simulink model "SEPIC_PhysicalModel_FMU"  (R2024b)
settings: Solver=VariableStepAuto  StartTime=0.0  StopTime=10.0  RelTol=1e-3
undefined symbols (not defined in the file): D1_Vf, FPWM1, FPWM1_Volt, M1_Vth, PR1_Res, psu_V, R9_Res
libraries: fl_lib x10, ee_lib x8, nesl_utility x7, simulink x1
settings Model: DataDictionary=GlobalDataD_SEPIC_PhysicalCircuit.sldd  ExtModeTrigDuration=100  Creator=vlenzi  LastModifiedBy=vlenzi
settings DataIOCC: StateSaveName=tmp_raccel_xout
settings OptimizationCC: EfficientMapNaN2IntZero=off
settings DebuggingCC: ModelReferenceSymbolNameMessage=none
settings HardwareCC: TargetBitPerPointer=64  TargetBitPerSizeT=64  TargetBitPerPtrDiffT=64  TargetLongLongMode=on  TargetIntDivRoundTo=Zero  TargetEndianess=LittleEndian  TargetWordSize=64  TargetHWDeviceType=MATLAB Host  ProdEqTarget=off
settings RTWCC: SystemTargetFile=raccel.tlc  TemplateMakefile=raccel_default_tmf  RTWVerbose=off  RTWUseSimCustomCode=on  CustomBLASCallback=coder.internal.blas.MATLABBLASCallback
settings CodeAppCC: GenerateComments=off  MaxIdLength=128  MangleLength=10  SimulinkBlockComments=off
settings RaccelTargetCC: TargetLangStandard=C99 (ISO)  InstructionSetFMA=off  OptimizeReductions=off  LogToMDFFile=off  ENABLE_SLEXEC_SSBRIDGE=1  RTWCAPIParams=on  RTWCAPIRootIO=on

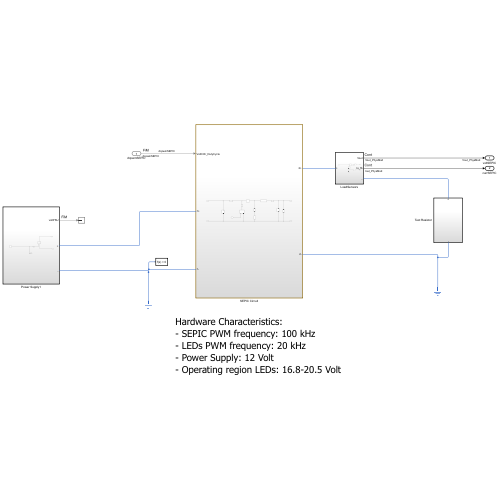
[thumbnail: Simulink's stored preview of the top-level diagram]
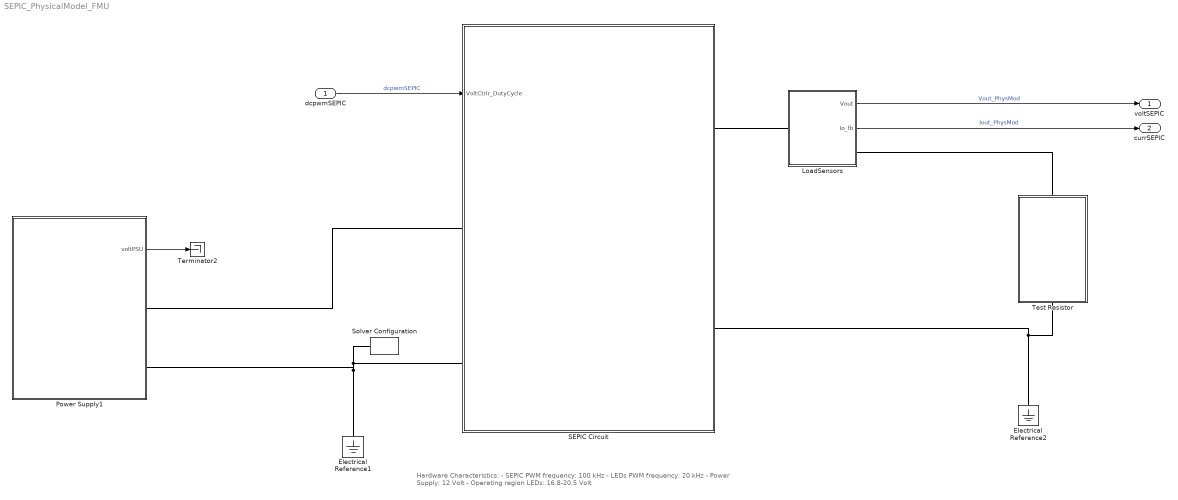
== system SEPIC_PhysicalModel_FMU ==
  note: Hardware Characteristics:
      | - SEPIC PWM frequency: 100 kHz
      | - LEDs PWM frequency: 20 kHz
      | - Power Supply: 12 Volt
      | - Operating region LEDs: 16.8-20.5 Volt
  dcpwmSEPIC : Inport  OutDataTypeStr=double  Unit=1  PortDimensions=1
  Electrical Reference1 : fl_lib/Electrical/Electrical Elements/Electrical Reference
  Electrical Reference2 : fl_lib/Electrical/Electrical Elements/Electrical Reference
  LoadSensors : Subsystem
  Power Supply1 : Subsystem  VariantControl=PowerSupply
  SEPIC Circuit : Subsystem
  Solver Configuration : nesl_utility/Solver Configuration  PhysicalDomain=network_engine_domain  SubClassName=solver  LeftPortType=input  RightPortType=generic  Tones=[]  Harmonics=[]  SimulateNoise=off  Profile=off  UseLocalSampling=off  EnableSwitchedLinearOptims=on  FrequencyDomain=off  UseCCode=off  RelTol=0.001  AbsTol=1e-06  MinStep=1e-09  ToWorkspace=off  RevertToSquareIcSolve=off  NumHomotopyIterations=100  PhasorMode=off  PhasorModeNumHarmonics=1  ConsistencySolver=NEWTON_XTOL_AFTER_FTOL  IndexReductionMethod=DerivativeReplacement  DoDC=off  ResidualTolerance=1e-9  ConsistencyTolSource=GLOBAL  ConsistencyAbsTol=0.001  ConsistencyRelTol=0.001  ConsistencyTolFactor=0.001  UseLocalSolver=off  LocalSolverChoice=NE_BACKWARD_EULER_ADVANCER  ResolveIndetEquations=on  FunctionEvalNumThread=1  LocalSolverSampleTime=2e-7  DoFixedCost=off  MaxNonlinIter=2  MaxModeIter=2  ComputeImpulses=off  ImpulseIterations=2  LinearAlgebra=Sparse  LinearAlgebraNumThread=0  EquationFormulation=NE_TIME_EF  DelaysMemoryBudget=1024  AutomaticFiltering=on  FilteringTimeConstant=0.001  PartitionStorageMethod=AS_NEEDED  PartitionMemoryBudget=1024  PartitionMethod=ROBUST  MultibodyUseLocalSolver=off  MultibodyLocalSolverChoice=ODE1  MultibodyLocalSolverSampleTime=0.001
  Terminator2 : Terminator
  Test Resistor : Subsystem  VariantControl=Resistor
  voltSEPIC : Outport  OutDataTypeStr=double  Unit=V  PortDimensions=1  VectorParamsAs1DForOutWhenUnconnected=off
  currSEPIC : Outport  Port=2  OutDataTypeStr=double  Unit=mA  PortDimensions=1  VectorParamsAs1DForOutWhenUnconnected=off
  wires:
  dcpwmSEPIC/1 -> SEPIC Circuit/1(VoltCtrlr_DutyCycle)  "dcpwmSEPIC"
  LoadSensors/1(Vout) -> voltSEPIC/1  "Vout_PhysMod"
  Power Supply1/1(voltPSU) -> Terminator2/1
  LoadSensors/2(Io_fb) -> currSEPIC/1  "Iout_PhysMod"
  connections:
  Power Supply1/RConn1 -- SEPIC Circuit/LConn1
  Solver Configuration/RConn1 -- Power Supply1/RConn2 -- Electrical Reference1/LConn1 -- SEPIC Circuit/LConn2
  SEPIC Circuit/RConn1 -- LoadSensors/LConn1
  Electrical Reference2/LConn1 -- SEPIC Circuit/RConn2 -- Test Resistor/RConn1
  Test Resistor/LConn1 -- LoadSensors/RConn1

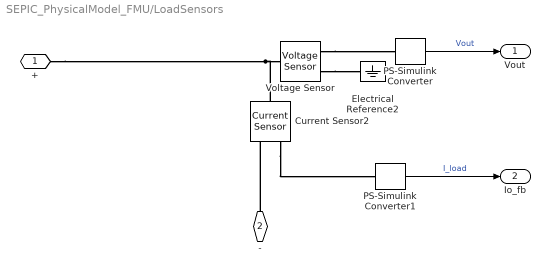
== system SEPIC_PhysicalModel_FMU/LoadSensors ==
  Current Sensor2 : fl_lib/Electrical/Electrical Sensors/Current Sensor
  Electrical Reference2 : fl_lib/Electrical/Electrical Elements/Electrical Reference
  PS-Simulink Converter : nesl_utility/PS-Simulink Converter  PhysicalDomain=network_engine_domain  SubClassName=ps_output  LeftPortType=input  RightPortType=output  PseudoPeriodic=off  Frequencies=[]  VectorFormat=1-D array  Unit=V  AffineConversion=off
  PS-Simulink Converter1 : nesl_utility/PS-Simulink Converter  PhysicalDomain=network_engine_domain  SubClassName=ps_output  LeftPortType=input  RightPortType=output  PseudoPeriodic=off  Frequencies=[]  VectorFormat=1-D array  Unit=mA  AffineConversion=off
  Voltage Sensor : fl_lib/Electrical/Electrical Sensors/Voltage Sensor
  + : PMIOPort  Side=Left
  - : PMIOPort  Port=2  Side=Right
  Vout : Outport  VectorParamsAs1DForOutWhenUnconnected=off
  Io_fb : Outport  Port=2  VectorParamsAs1DForOutWhenUnconnected=off
  wires:
  PS-Simulink Converter1/1 -> Io_fb/1  "I_load"
  PS-Simulink Converter/1 -> Vout/1  "Vout"
  connections:
  Voltage Sensor/RConn1 -- PS-Simulink Converter/LConn1
  Voltage Sensor/RConn2 -- Electrical Reference2/LConn1
  Current Sensor2/LConn1 -- Voltage Sensor/LConn1 -- +/RConn1
  Current Sensor2/RConn1 -- PS-Simulink Converter1/LConn1
  -/RConn1 -- Current Sensor2/RConn2

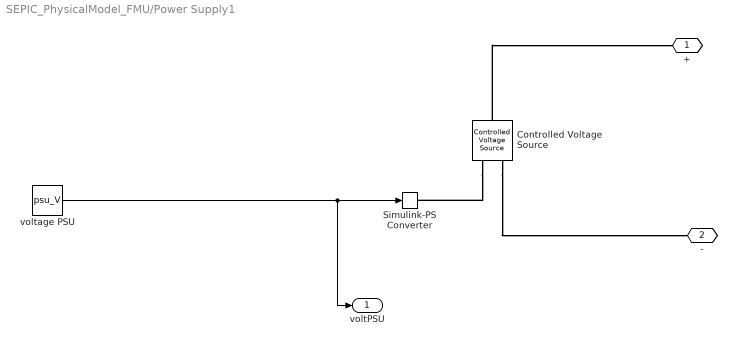
== system SEPIC_PhysicalModel_FMU/Power Supply1 ==
  Controlled Voltage Source : fl_lib/Electrical/Electrical Sources/Controlled Voltage Source
  Simulink-PS Converter : nesl_utility/Simulink-PS Converter  PhysicalDomain=network_engine_domain  SubClassName=ps_input  LeftPortType=input  RightPortType=output  PseudoPeriodic=off  Frequencies=[]  NoiseDistribution=none  NoiseParameters=[]  Unit=V  AffineConversion=off  FilteringAndDerivatives=filter  SimscapeFilterOrder=1  InputFilterTimeConstant=0.001  UdotUserProvided=0
  voltage PSU : Constant  Value=psu_V  OutDataTypeStr=double  SampleTime=-1
  + : PMIOPort  Side=Right
  - : PMIOPort  Port=2  Side=Right
  voltPSU : Outport  Unit=V  VectorParamsAs1DForOutWhenUnconnected=off
  wires:
  voltage PSU/1 -> voltPSU/1, Simulink-PS Converter/1
  connections:
  Controlled Voltage Source/RConn2 -- -/RConn1
  Controlled Voltage Source/RConn1 -- Simulink-PS Converter/RConn1
  Controlled Voltage Source/LConn1 -- +/RConn1

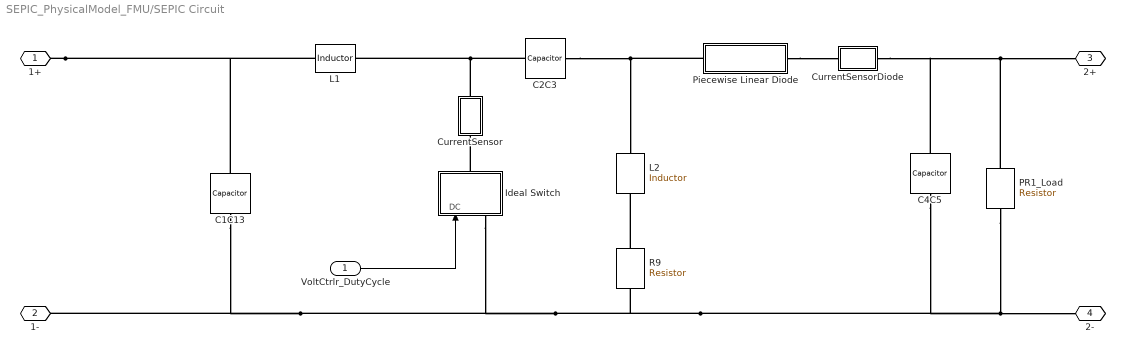
== system SEPIC_PhysicalModel_FMU/SEPIC Circuit ==
  VoltCtrlr_DutyCycle : Inport  Unit=1  PortDimensions=1
  C1C13 : ee_lib/Passive/Capacitor  cap_option=ee.enum.passive.capacitor.capOption.const  c=C1C13_Cap uF  Cvec=[1e-05, 1e-06] F  Vvec=[0, 10] V  CV_table_symmetry=1  f_vec=[1, 10] kHz  DFext_vec=[.8, 1.2]  enable_C_tol=0  averaging_period=0 s  C_tol=C1C13_Tol  tol_distribution=1  nSigma=4  r=1e-6 Ohm  g=0 1/Ohm  enable_operating_limits=0  operating_limit_action=2  max_working_voltage_range=[-25, 25] V  power_rating=1 W  maxTemperature=85 degC  thermalEnable=false  thermalMass=1 J/K  fault_action=simscape.enum.assert.action.none  t_fault=1 s  i_specify=off  i_priority=None  i=0 A  i_nominal_specify=off  i_nominal_value=1  i_nominal_unit=A  v_specify=off  v_priority=High  v=psu_V V  v_nominal_specify=off  v_nominal_value=1  v_nominal_unit=V  vc_specify=off  vc_priority=High  vc=psu_V V  vc_nominal_specify=off  vc_nominal_value=1  vc_nominal_unit=V  T_specify=off  T_priority=None  T=298.15 K  T_nominal_specify=off  T_nominal_value=1  T_nominal_unit=K
  C2C3 : ee_lib/Passive/Capacitor  cap_option=ee.enum.passive.capacitor.capOption.const  c=C2C3_Cap uF  Cvec=[1e-05, 1e-06] F  Vvec=[0, 10] V  CV_table_symmetry=1  f_vec=[1, 10] kHz  DFext_vec=[.8, 1.2]  enable_C_tol=0  averaging_period=0 s  C_tol=C2C3_Tol  tol_distribution=1  nSigma=4  r=1e-6 Ohm  g=0 1/Ohm  enable_operating_limits=0  operating_limit_action=2  max_working_voltage_range=[-25, 25] V  power_rating=1 W  maxTemperature=85 degC  thermalEnable=false  thermalMass=1 J/K  fault_action=simscape.enum.assert.action.none  t_fault=1 s  i_specify=off  i_priority=None  i=0 A  i_nominal_specify=off  i_nominal_value=1  i_nominal_unit=A  v_specify=off  v_priority=High  v=psu_V V  v_nominal_specify=off  v_nominal_value=1  v_nominal_unit=V  vc_specify=off  vc_priority=High  vc=psu_V V  vc_nominal_specify=off  vc_nominal_value=1  vc_nominal_unit=V  T_specify=off  T_priority=None  T=298.15 K  T_nominal_specify=off  T_nominal_value=1  T_nominal_unit=K
  C4C5 : ee_lib/Passive/Capacitor  cap_option=ee.enum.passive.capacitor.capOption.const  c=C4C5_Cap uF  Cvec=[1e-05, 1e-06] F  Vvec=[0, 10] V  CV_table_symmetry=1  f_vec=[1, 10] kHz  DFext_vec=[.8, 1.2]  enable_C_tol=0  averaging_period=0 s  C_tol=C4C5_Tol  tol_distribution=1  nSigma=4  r=1e-6 Ohm  g=0 1/Ohm  enable_operating_limits=0  operating_limit_action=2  max_working_voltage_range=[-25, 25] V  power_rating=1 W  maxTemperature=85 degC  thermalEnable=false  thermalMass=1 J/K  fault_action=simscape.enum.assert.action.none  t_fault=1 s  i_specify=off  i_priority=None  i=0 A  i_nominal_specify=off  i_nominal_value=1  i_nominal_unit=A  v_specify=off  v_priority=High  v=desiredVoltage_Param V  v_nominal_specify=off  v_nominal_value=1  v_nominal_unit=V  vc_specify=off  vc_priority=High  vc=desiredVoltage_Param V  vc_nominal_specify=off  vc_nominal_value=1  vc_nominal_unit=V  T_specify=off  T_priority=None  T=298.15 K  T_nominal_specify=off  T_nominal_value=1  T_nominal_unit=K
  CurrentSensor : Subsystem
  CurrentSensorDiode : Subsystem
  Ideal Switch : Subsystem  VariantControl=Ideal
  L1 : ee_lib/Passive/Inductor  l=L1_Ind uH  enable_L_tol=0  L_tol=L1_Tol  tol_distribution=1  nSigma=4  r=L1_Res Ohm  g=0 1/Ohm  enable_operating_limits=0  operating_limit_action=2  max_working_current=1 A  power_rating=1 W  fault_action=simscape.enum.assert.action.none  t_fault=1 s  i_L_specify=off  i_L_priority=High  i_L=0 A  i_L_nominal_specify=off  i_L_nominal_value=1  i_L_nominal_unit=A
  L2 : ee_lib/Passive/Inductor  l=L2_Ind uH  enable_L_tol=0  L_tol=L2_Tol  tol_distribution=1  nSigma=4  r=L2_Res Ohm  g=0 1/Ohm  enable_operating_limits=0  operating_limit_action=2  max_working_current=1 A  power_rating=1 W  fault_action=simscape.enum.assert.action.none  t_fault=1 s  i_L_specify=off  i_L_priority=High  i_L=0 A  i_L_nominal_specify=off  i_L_nominal_value=1  i_L_nominal_unit=A
  PR1_Load : ee_lib/Passive/Resistor  R=PR1_Res Ohm  enable_R_tol=0  R_tol=PR1_Tol  tol_distribution=1  nSigma=4  enable_operating_limits=0  operating_limit_action=2  power_rating=1 W  max_working_voltage=100 V  noise_mode=0  Tdevice=25 degC  sample_time=1e-3 s  repeatability=1  user_seed=0  auto_seed=1185518679  fault_action=simscape.enum.assert.action.none  t_fault=1 s  power_derating_T1=70 degC  power_derating_T2=155 degC  operating_temperature_range_vec=[-50, 150] degC  alpha=3.93e-3 1/K  Tmeas=25 degC  thermal_mass=100 J/K  temperature_specify=off  temperature_priority=High  temperature=298.15 K  temperature_nominal_specify=off  temperature_nominal_value=1  temperature_nominal_unit=K
  Piecewise Linear Diode : Subsystem  VariantControl=PiecewiseLinear
  R9 : ee_lib/Passive/Resistor  R=R9_Res Ohm  enable_R_tol=2  R_tol=R9_Tol  tol_distribution=1  nSigma=4  enable_operating_limits=0  operating_limit_action=2  power_rating=1 W  max_working_voltage=100 V  noise_mode=0  Tdevice=25 degC  sample_time=1e-3 s  repeatability=1  user_seed=0  auto_seed=2919300768  fault_action=simscape.enum.assert.action.none  t_fault=1 s  power_derating_T1=70 degC  power_derating_T2=155 degC  operating_temperature_range_vec=[-50, 150] degC  alpha=3.93e-3 1/K  Tmeas=25 degC  thermal_mass=100 J/K  temperature_specify=off  temperature_priority=High  temperature=298.15 K  temperature_nominal_specify=off  temperature_nominal_value=1  temperature_nominal_unit=K
  1+ : PMIOPort  Side=Left
  1- : PMIOPort  Port=2  Side=Left
  2+ : PMIOPort  Port=3  Side=Right
  2- : PMIOPort  Port=4  Side=Right
  wires:
  VoltCtrlr_DutyCycle/1 -> Ideal Switch/1(DC)
  connections:
  C2C3/LConn1 -- L1/RConn1 -- CurrentSensor/LConn1
  PR1_Load/LConn1 -- 2+/RConn1 -- CurrentSensorDiode/RConn1 -- C4C5/LConn1
  C2C3/RConn1 -- Piecewise Linear Diode/LConn1 -- L2/LConn1
  PR1_Load/RConn1 -- 2-/RConn1 -- C4C5/RConn1 -- R9/RConn1 -- Ideal Switch/LConn1 -- 1-/RConn1 -- C1C13/RConn1
  1+/RConn1 -- C1C13/LConn1 -- L1/LConn1
  Ideal Switch/RConn1 -- CurrentSensor/RConn1
  R9/LConn1 -- L2/RConn1
  Piecewise Linear Diode/RConn1 -- CurrentSensorDiode/LConn1

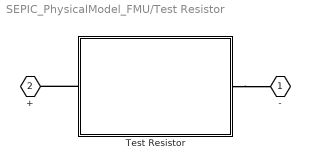
== system SEPIC_PhysicalModel_FMU/Test Resistor ==
  Test Resistor : Subsystem  VariantControl=Resistor  mask(Test Resistor){R_load=101.1, R_tol=1}
      mask prompts: R_load "Load Resistance [ohm]"; R_tol "Tolerance [%]"
      mask help: Test resistor with Load in the name, so that it can be triggered by ee_getEfficiency function.
  - : PMIOPort  Side=Right
  + : PMIOPort  Port=2  Side=Left
  connections:
  Test Resistor/LConn1 -- +/RConn1
  Test Resistor/RConn1 -- -/RConn1

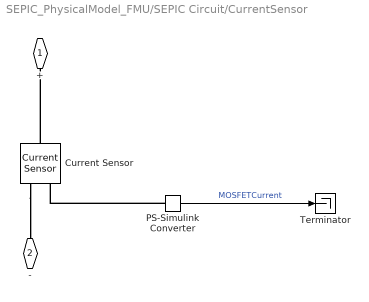
== system SEPIC_PhysicalModel_FMU/SEPIC Circuit/CurrentSensor ==
  Current Sensor : fl_lib/Electrical/Electrical Sensors/Current Sensor
  PS-Simulink Converter : nesl_utility/PS-Simulink Converter  PhysicalDomain=network_engine_domain  SubClassName=ps_output  LeftPortType=input  RightPortType=output  PseudoPeriodic=off  Frequencies=[]  VectorFormat=1-D array  Unit=A  AffineConversion=off
  Terminator : Terminator
  + : PMIOPort  Side=Left
  - : PMIOPort  Port=2  Side=Right
  wires:
  PS-Simulink Converter/1 -> Terminator/1  "MOSFETCurrent"
  connections:
  Current Sensor/LConn1 -- +/RConn1
  PS-Simulink Converter/LConn1 -- Current Sensor/RConn1
  Current Sensor/RConn2 -- -/RConn1

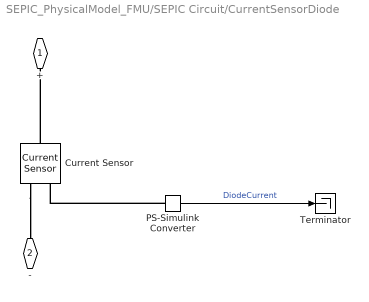
== system SEPIC_PhysicalModel_FMU/SEPIC Circuit/CurrentSensorDiode ==
  Current Sensor : fl_lib/Electrical/Electrical Sensors/Current Sensor
  PS-Simulink Converter : nesl_utility/PS-Simulink Converter  PhysicalDomain=network_engine_domain  SubClassName=ps_output  LeftPortType=input  RightPortType=output  PseudoPeriodic=off  Frequencies=[]  VectorFormat=1-D array  Unit=A  AffineConversion=off
  Terminator : Terminator
  + : PMIOPort  Side=Left
  - : PMIOPort  Port=2  Side=Right
  wires:
  PS-Simulink Converter/1 -> Terminator/1  "DiodeCurrent"
  connections:
  Current Sensor/RConn2 -- -/RConn1
  PS-Simulink Converter/LConn1 -- Current Sensor/RConn1
  Current Sensor/LConn1 -- +/RConn1

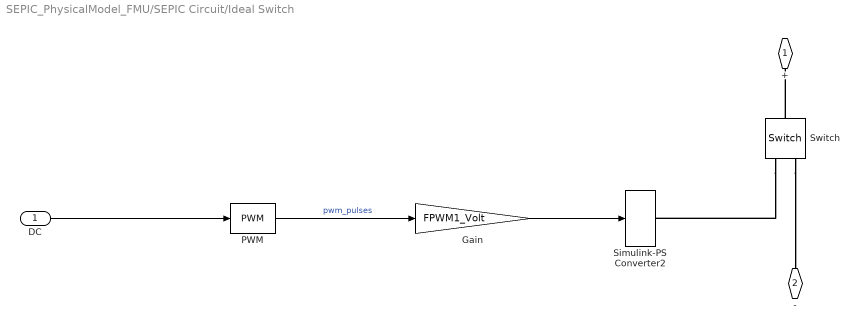
== system SEPIC_PhysicalModel_FMU/SEPIC Circuit/Ideal Switch ==
  DC : Inport
  Gain : Gain  Gain=FPWM1_Volt
  PWM : simulink/Discontinuities/PWM  DisableCoverage=on  Period=1/double(FPWM1)  InitialDelay=0  DisallowZeroDutyCycle=off  RunAtFixedTimeIntervals=off  SampleTime=0.1
  Simulink-PS Converter2 : nesl_utility/Simulink-PS Converter  PhysicalDomain=network_engine_domain  SubClassName=ps_input  LeftPortType=input  RightPortType=output  PseudoPeriodic=off  Frequencies=[]  NoiseDistribution=none  NoiseParameters=[]  Unit=1  AffineConversion=off  FilteringAndDerivatives=provide  SimscapeFilterOrder=1  InputFilterTimeConstant=1e-7  UdotUserProvided=0
  Switch : fl_lib/Electrical/Electrical Elements/Switch  R_closed=S1_Rds Ohm  G_open=1e-6 1/Ohm  Threshold=M1_Vth  i_specify=off  i_priority=None  i=0 A  i_nominal_specify=off  i_nominal_value=1  i_nominal_unit=A  v_specify=off  v_priority=None  v=0 V  v_nominal_specify=off  v_nominal_value=1  v_nominal_unit=V
  + : PMIOPort  Side=Right
  - : PMIOPort  Port=2  Side=Left
  wires:
  Gain/1 -> Simulink-PS Converter2/1
  PWM/1 -> Gain/1  "pwm_pulses"
  DC/1 -> PWM/1
  connections:
  Switch/LConn1 -- +/RConn1
  Switch/RConn1 -- Simulink-PS Converter2/RConn1
  Switch/RConn2 -- -/RConn1

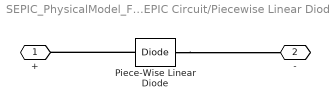
== system SEPIC_PhysicalModel_FMU/SEPIC Circuit/Piecewise Linear Diode ==
  Piece-Wise Linear Diode : fl_lib/Electrical/Electrical Elements/Diode  Vf=D1_Vf(1) V  Ron=D1_Rs Ohm  Goff=1e-8 1/Ohm  i_specify=off  i_priority=None  i=0 A  i_nominal_specify=off  i_nominal_value=1  i_nominal_unit=A  v_specify=off  v_priority=None  v=0 V  v_nominal_specify=off  v_nominal_value=1  v_nominal_unit=V
  + : PMIOPort  Side=Left
  - : PMIOPort  Port=2  Side=Right
  connections:
  Piece-Wise Linear Diode/LConn1 -- +/RConn1
  Piece-Wise Linear Diode/RConn1 -- -/RConn1

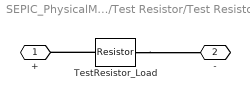
== system SEPIC_PhysicalModel_FMU/Test Resistor/Test Resistor ==
  TestResistor_Load : ee_lib/Passive/Resistor  R=R_load Ohm  enable_R_tol=0  R_tol=R_tol  tol_distribution=1  nSigma=4  enable_operating_limits=0  operating_limit_action=2  power_rating=1 W  max_working_voltage=100 V  noise_mode=0  Tdevice=25 degC  sample_time=1e-3 s  repeatability=1  user_seed=0  auto_seed=3536724442  fault_action=simscape.enum.assert.action.none  t_fault=1 s  power_derating_T1=70 degC  power_derating_T2=155 degC  operating_temperature_range_vec=[-50, 150] degC  alpha=3.93e-3 1/K  Tmeas=25 degC  thermal_mass=100 J/K  temperature_specify=off  temperature_priority=High  temperature=298.15 K  temperature_nominal_specify=off  temperature_nominal_value=1  temperature_nominal_unit=K
  + : PMIOPort  Side=Left
  - : PMIOPort  Port=2  Side=Right
  connections:
  TestResistor_Load/LConn1 -- +/RConn1
  TestResistor_Load/RConn1 -- -/RConn1
